simulink model "lb231_usrp_tx_ppm"  (R2018b)
settings: Solver=VariableStepAuto  StartTime=0.0  StopTime=inf  RelTol=1e-3
libraries: commsdrhw_v2 x1, dspsrcs4 x1
settings Model: Creator=Григорий Фокин  LastModifiedBy=Григорий Фокин
settings SFSimCC: SimUseLocalCustomCode=off
settings RTWCC: RTWUseLocalCustomCode=off
settings CodeAppCC: StateflowObjectComments=on

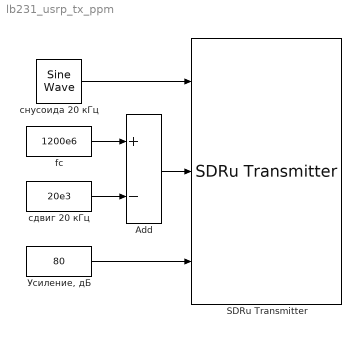
== system lb231_usrp_tx_ppm ==
  Add : Sum  Inputs=+-
  SDRu Transmitter : commsdrhw_v2/SDRu Transmitter  rxtx=tx  initializeIPAddress=0  devMap=0  USRP2_IP=192.168.10.2  USRP_IP_X300=192.168.10.2  USRP_IP_X310=192.168.10.2  USRP_serialNumB200=No devices found  USRP_serialNumB210=F4E642  platform=B210  prevPlatform=B210  lastIPAddressPopup=192.168.10.2  USRP_ID=F4E642  LastIPAddress=192.168.10.2  ChannelMapping=1  centerFrequencySrc=Input port  centerFrequency=2.45e9  loOffsetSrc=Dialog  loOffset=0  gainSrc=Input port  gain=8  PPSSource=Internal  clockSource=Internal  masterClkRateParam=6000000  masterClkRateB200=32e6  masterClkRateB210=6e6  masterClkRateX300=200e6  masterClkRateX310=200e6  decimInterpSrc=Dialog  decimInterp=30  USRP2_IP_NUM=[70 52 69 54 52 50]  frameLength=362  TransportDataType=int16  outputDatatype=Same as transport data type  overrunUnderrunPort=off  sampleTime=1  dboardInfo=|  HOST_DATA_PORT=30000  HOST_CONTROL_PORT=30001  USRP2_DATA_PORT=32769  USRP2_CONTROL_PORT=32768  bufferMode=Continuous streaming  EnableBurstMode=off  NumFramesInBurst=100
      | dbid: 0
      |           dbName: 'no db found'
      |          freqMin: 0
      |          freqMax: 0
      |          gainMin: 0
      |          gainMax: 0
      |     gainStepSize: 0
      settings: SourceProductName=Communications System Toolbox Support Package for USRP(R) Radio  SourceProductBaseCode=USRP
  fc : Constant  Value=1200e6
  "Усиление, дБ" : Constant  Value=80
  сдвиг 20 кГц : Constant  Value=20e3
  снусоида 20 кГц : dspsrcs4/Sine Wave  Amplitude=1  Frequency=20e3  Phase=0  SampleMode=Discrete  OutComplex=Complex  CompMethod=Trigonometric fcn  TableSize=Speed  SampleTime=1/200e3  SamplesPerFrame=1  ResetState=Restart at time zero  OutputFrames=off  dataType=double  wordLen=16  udDataType=sfix(16)  fracBitsMode=Best precision  numFracBits=15  OutDataTypeStr=double  LastOutDataTypeStr=double
  wires:
  Add/1 -> SDRu Transmitter/2
  fc/1 -> Add/1
  сдвиг 20 кГц/1 -> Add/2
  "Усиление, дБ"/1 -> SDRu Transmitter/3
  снусоида 20 кГц/1 -> SDRu Transmitter/1
